simulink model "crane_simulink_a1"  (R2017a)
settings: Solver=VariableStepAuto  StartTime=0.0  StopTime=tf  MaxStep=maxstep  RelTol=tol
values from neighbouring files (symbols this model uses):
  C = mp*Lpcg + mw*Lwcg    [crane_script.m]
  J = mp*Lp^2/12 + mp*Lpcg^2 + (1/2)*mw*(dw/2)^2 + mw*Lwcg^2    [crane_script.m]
  k = g*(mp*Lpcg+mw*Lwcg)    [crane_script.m]
settings Model: Creator=eckelsjd  LastModifiedBy=eckelsjd

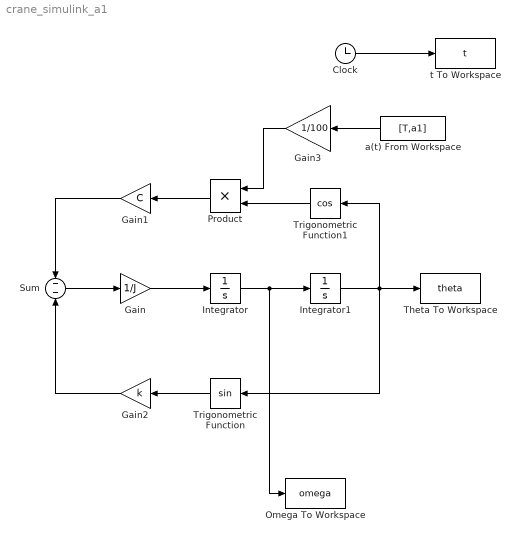
== system crane_simulink_a1 ==
  Clock : Clock
  Gain : Gain  Gain=1/J
  Gain1 : Gain  Gain=C
  Gain2 : Gain  Gain=k
  Gain3 : Gain  Gain=1/100
  Integrator : Integrator
  Integrator1 : Integrator
  Omega To Workspace : ToWorkspace  VariableName=omega  SampleTime=-1
  Product : Product
  Sum : Sum  Inputs=--
  Theta To Workspace : ToWorkspace  VariableName=theta  SampleTime=-1
  Trigonometric Function : Trigonometry
  Trigonometric Function1 : Trigonometry  Operator=cos
  a(t) From Workspace : FromWorkspace  VariableName=[T,a1]  SampleTime=0  OutputAfterFinalValue=Setting to zero
  t To Workspace : ToWorkspace  VariableName=t  SampleTime=-1
  wires:
  Sum/1 -> Gain/1
  Gain/1 -> Integrator/1
  Integrator/1 -> Omega To Workspace/1, Integrator1/1
  Integrator1/1 -> Trigonometric Function/1, Theta To Workspace/1, Trigonometric Function1/1
  Trigonometric Function1/1 -> Product/2
  Product/1 -> Gain1/1
  Gain1/1 -> Sum/1
  Trigonometric Function/1 -> Gain2/1
  Gain2/1 -> Sum/2
  Clock/1 -> t To Workspace/1
  a(t) From Workspace/1 -> Gain3/1
  Gain3/1 -> Product/1
